simulink model "dsp232311226"  (R2026a)
settings: Solver=FixedStepDiscrete  FixedStep=0.001
undefined symbols (not defined in the file): depth
libraries: simulink x1, dspfdesign x1
settings Model: Creator=HP  LastModifiedBy=HP

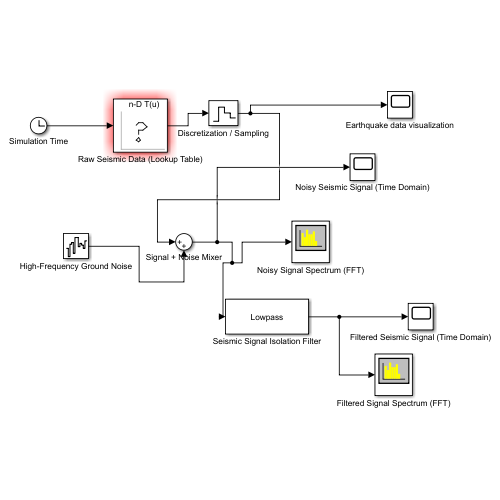
[thumbnail: Simulink's stored preview of the top-level diagram]
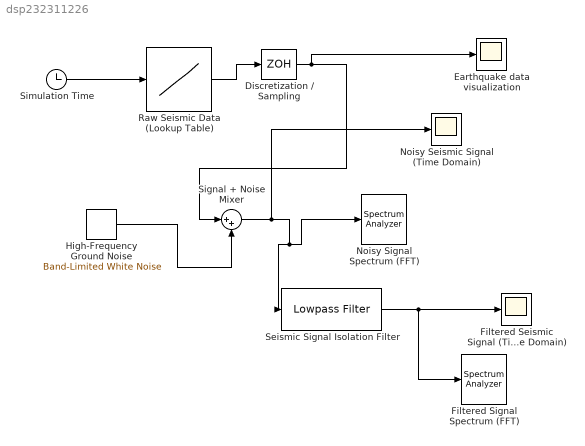
== system dsp232311226 ==
  Discretization / Sampling : ZeroOrderHold  SampleTime=0.001
  Earthquake data visualization : Scope
      settings: ActiveDisplayYMinimum=-210.53612429563171  ActiveDisplayYMaximum=214.05642824089171
  Filtered Seismic Signal (Time Domain) : Scope
      settings: ActiveDisplayYMinimum=-122.68189786468912  ActiveDisplayYMaximum=185.805598551134  DataLoggingVariableName=ScopeData2
  Filtered Signal Spectrum (FFT) : SpectrumAnalyzer  WindowPosition=[916.000000,499.000000,256.000000,206.000000,]  ScopeFrameLocation=window  WindowInvariantSamplesPerUpdate=on  YLimits=[-9.0582 75.4259]
  High-Frequency Ground Noise : simulink/Sources/Band-Limited White Noise  Cov=0.1  Ts=0.001  seed=[23341]
  Noisy Seismic Signal (Time Domain) : Scope
      settings: ActiveDisplayYMinimum=-142.9676947786636  ActiveDisplayYMaximum=208.66505795388898
  Noisy Signal Spectrum (FFT) : SpectrumAnalyzer  WindowPosition=[613.000000,509.000000,279.000000,200.000000,]  ScopeFrameLocation=window  WindowInvariantSamplesPerUpdate=on  YLimits=[7.6404 73.1876]
  Raw Seismic Data (Lookup Table) : Lookup_n-D  NumberOfTableDimensions=1  BreakpointsForDimension1=1:40  Table=depth  InternalRulePriority=Speed  RndMeth=Simplest
  Seismic Signal Isolation Filter : dspfdesign/Lowpass Filter  FilterType=FIR  DesignForMinimumOrder=on  FilterOrder=50  PassbandFrequency=10  StopbandFrequency=15  PassbandRipple=0.1  StopbandAttenuation=80  SampleRateMode=Specify on dialog  SampleRate=1000  SimulateUsing=Interpreted execution  roundingMode=Floor  coeffsDataTypeStr=fixdt(1,16)
  Signal + Noise Mixer : Sum  Inputs=|++
  Simulation Time : Clock
  wires:
  Simulation Time/1 -> Raw Seismic Data (Lookup Table)/1
  High-Frequency Ground Noise/1 -> Signal + Noise Mixer/2
  Signal + Noise Mixer/1 -> Seismic Signal Isolation Filter/1, Noisy Signal Spectrum (FFT)/1, Noisy Seismic Signal (Time Domain)/1
  Seismic Signal Isolation Filter/1 -> Filtered Signal Spectrum (FFT)/1, Filtered Seismic Signal (Time Domain)/1
  Raw Seismic Data (Lookup Table)/1 -> Discretization / Sampling/1
  Discretization / Sampling/1 -> Signal + Noise Mixer/1, Earthquake data visualization/1
